simulink model "ctrl_HSMBObserver"  (R2015a)
settings: Solver=ode3  StartTime=0.0  StopTime=inf  FixedStep=0.01  RelTol=1e-3
values from neighbouring files (symbols this model uses):
  C = [C1;C2;C3;C4;C5;C6]    [initfile.m]    (also in thrustallocationQuadraticFixed.m)
  D = 3.0/100    (= 0.03)    [initfile.m]    (also in thrustallocationQuadraticFixed.m = 0.0411111111111)
  eps_c = 5    [initfile.m]
  epsilon = 0.5    [initfile.m]    (also in thrustallocationPseudo.m = u(10); thrustallocationQuadraticFixed.m = u(10))
  hd = c2d(H1,0.01,'foh')    [initfile.m]
  hd2 = c2d(H2,0.01,'zoh')    [initfile.m]
  I_s = 25000 /747225    (= 0.0334571246947)    [initfile.m]
  k_cc = 1    [initfile.m]
  K_omega = 0.3    [initfile.m]
  K_q1f = 0.0113    [initfile.m]
  K_q1r = K_q1f    (= 0.0113)    [initfile.m]
  K_q2f = 0.0117    [initfile.m]
  K_q2r = K_q2f    (= 0.0117)    [initfile.m]
  K_q3f = 0.0113    [initfile.m]
  K_q3r = K_q3f    (= 0.0113)    [initfile.m]
  K_q4f = 0.0169    [initfile.m]
  K_q4r = K_q4f    (= 0.0169)    [initfile.m]
  K_q5f = 0.0144    [initfile.m]
  K_q5r = K_q5f    (= 0.0144)    [initfile.m]
  K_q6f = 0.0168    [initfile.m]
  K_q6r = K_q6f    (= 0.0168)    [initfile.m]
  K_T1f = 0.3763    [initfile.m]
  K_T1r = K_T1f    (= 0.3763)    [initfile.m]
  K_T2f = 0.3901    [initfile.m]
  K_T2r = K_T2f    (= 0.3901)    [initfile.m]
  K_T3f = 0.3776    [initfile.m]
  K_T3r = K_T3f    (= 0.3776)    [initfile.m]
  K_T4f = 0.5641    [initfile.m]
  K_T4r = K_T4f    (= 0.5641)    [initfile.m]
  K_T5f = 0.4799    [initfile.m]
  K_T5r = K_T5f    (= 0.4799)    [initfile.m]
  K_T6f = 0.5588    [initfile.m]
  K_T6r = K_T6f    (= 0.5588)    [initfile.m]
  Kp = 3.3    [initfile.m]
  Max_Acceleration = 5    [initfile.m]
  Max_rotation = 12*sqrt(lambda)    [initfile.m]
  Max_thrust = 1.5    [initfile.m]
  Min_thrust = -0.8    [initfile.m]
  n_c = 5    [initfile.m]
  n_max = 152    [initfile.m]
  p_cc = 0.5    [initfile.m]
  pwm_thr1_backward = coeffvalues(ForceToPWM)    [initfile.m]
  pwm_thr1_forward = coeffvalues(ForceToPWM)    [initfile.m]
  pwm_thr2_backward = coeffvalues(ForceToPWM)    [initfile.m]
  pwm_thr2_forward = coeffvalues(ForceToPWM)    [initfile.m]
  pwm_thr3_backward = coeffvalues(ForceToPWM)    [initfile.m]
  pwm_thr3_forward = coeffvalues(ForceToPWM)    [initfile.m]
  pwm_thr4_backward = coeffvalues(ForceToPWM)    [initfile.m]
  pwm_thr4_forward = coeffvalues(ForceToPWM)    [initfile.m]
  pwm_thr5_backward = coeffvalues(ForceToPWM)    [initfile.m]
  pwm_thr5_forward = coeffvalues(ForceToPWM)    [initfile.m]
  pwm_thr6_backward = coeffvalues(ForceToPWM)    [initfile.m]
  pwm_thr6_forward = coeffvalues(ForceToPWM)    [initfile.m]
  Q_f0 = 0.3    [initfile.m]
  r_cc = 4    [initfile.m]
  Rho = Rho_m    (= 1000)    [initfile.m]
  ts = [-1 0]    [thrustallocationPseudo.m]    (also in thrustallocationQuadraticFixed.m)
undefined symbols (not defined in the file or in its folder): AFB, arm, Att, Control, Damping, FaultDet, Glob, Grip, IntActionType, Mass, NPO, Obs, Omg0_min, Q_max, ReferenceMdl, Sensor, Sim, SwLogic, tau, Thruster, Thruster_lock
libraries: dspmtrx3 x14, marine_gnc x11, simulink_extras x9, dspstat3 x9, simulink x9, dsparch4 x6, dspspect3 x6
(part 2 of 7)

== system ctrl_HSMBObserver/Data Logging ==
  eta_m : Inport
  eta_m_ideal : Inport  Port=2
  rate_m : Inport  Port=3
  acc_m : Inport  Port=4
  tau_c : Inport  Port=5
  tau_ca : Inport  Port=6
  angle_c : Inport  Port=7
  thrust_c : Inport  Port=8
  pwm_c : Inport  Port=9
  reference : Inport  Port=10
  controller : Inport  Port=11
  observer : Inport  Port=12
  fault : Inport  Port=13
  hat_wp : Inport  Port=14
  logic : Inport  Port=15
  PDF_control : Inport  Port=16
  PDF_reference : Inport  Port=17
  Mux : Mux  Inputs=17
  To File : ToFile  Filename=HSMBObserver.mat  MatrixName=data  SampleTime=0.01
  wires:
  eta_m/1 -> Mux/1
  Mux/1 -> To File/1
  eta_m_ideal/1 -> Mux/2
  rate_m/1 -> Mux/3
  acc_m/1 -> Mux/4
  tau_c/1 -> Mux/5
  angle_c/1 -> Mux/7
  thrust_c/1 -> Mux/8
  pwm_c/1 -> Mux/9
  tau_ca/1 -> Mux/6
  reference/1 -> Mux/10
  controller/1 -> Mux/11
  observer/1 -> Mux/12
  fault/1 -> Mux/13
  hat_wp/1 -> Mux/14
  logic/1 -> Mux/15
  PDF_control/1 -> Mux/16
  PDF_reference/1 -> Mux/17

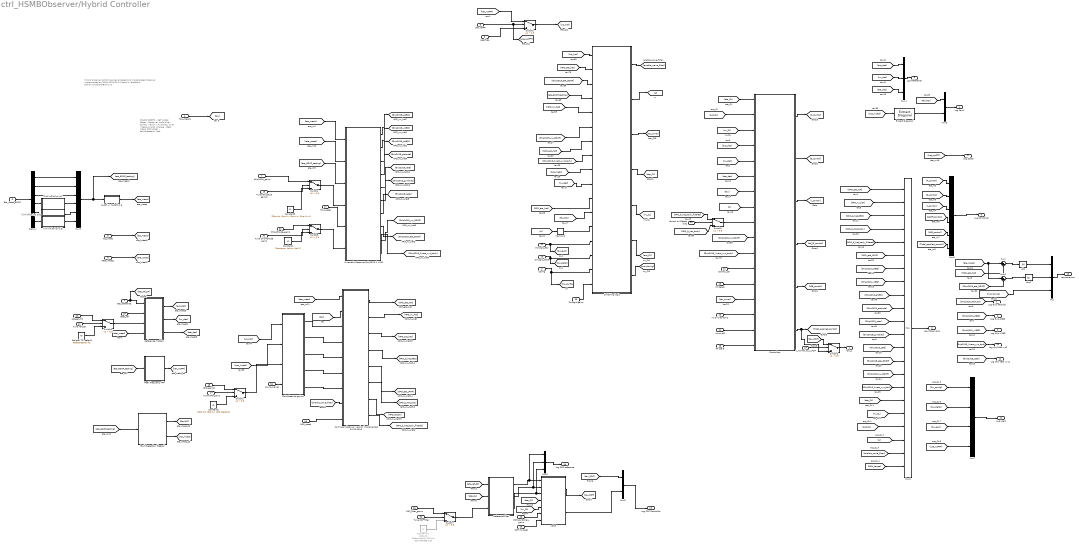
== system ctrl_HSMBObserver/Hybrid Controller ==
  note: Hybrid observer combining signal-based and model-based observer
      | Implemented on CSAD 2016-12-14
      | Astrid H. Brodtkorb astrid.h.brodtkorb@ntnu.no
  note: COLOR CODES:
      | 	- Ref model: Green
      | 	- Observer: Light blue
      | 	- Control: Yellow
      | 	- Hybrid/CL: Cyan
      | 	- Measurments: Orange
      | 	- Ideal meas: Dark green
      | 	- FaultDetection: Red
  Eta_reference : Inport
  Config : Inport  Port=2
  Eta_meas_6DOF : Inport  Port=3
  Tau_meas1 : Inport  Port=4
  Acc_meas : Inport  Port=5
  Rate_meas1 : Inport  Port=6
  Grip2015_gains : Inport  Port=7
  Use wpFFT : Inport  Port=8
  peakfreq : Inport  Port=9
  SwLogic_delta : Inport  Port=10
  SwLogic_eps : Inport  Port=11
  Control_par : Inport  Port=12
  Int Reset : Inport  Port=13
  Tune NPO gains : Inport  Port=14
  NPO_gains1 : Inport  Port=15
  Tune Grip2015 gains1 : Inport  Port=16
  Grip_reset : Inport  Port=17
  NPO_reset : Inport  Port=18
  reset_ref : Inport  Port=19
  ref_gen_TC : Inport  Port=20
  Tune ref gen : Inport  Port=21
  Normal or filtered bias : Inport  Port=22
  Int or bias comp : Inport  Port=23
  Int on/off : Inport  Port=24
  ref scale : Inport  Port=25
  PDF_filter_gains : Inport  Port=26
  u_normal_or_u_PDF : Inport  Port=27
  PDF_controller_gains : Inport  Port=28
  PDF int reset : Inport  Port=29
  Tune PDF filter : Inport  Port=30
  GripAttitude_gains : Inport  Port=31
  Tune GripAttitude gains : Inport  Port=32
  SwLogic.gains : Inport  Port=33
  K2_no_waves : Inport  Port=34
  6_dof --> 3_dof1,2,6 : Subsystem
  Abs : Abs
  Abs1 : Abs
  Calc observer gains1 : Subsystem  mask{lmb=Obs.NPO.lmb, k=Obs.NPO.k, zeta=Obs.NPO.damp}
      mask prompts: lmb "Control.VessObs.lmb{i}=lmb"; k "Control.VessObs.k{i}=k"; zeta "Control.VessObs.damp{i}=zeta"
  Constant1 : Constant  Value=[Att.sigma, Att.Kp, Att.Ki]
  Constant2 : Constant  Value=[NPO.K3, NPO.K4, NPO.scaleK2]
  Constant3 : Constant  Value=[Grip.Kp, Grip.Kv, Grip.Kxi, Grip.Kvvr]
  Controllers : Subsystem
  Demux : Demux  Outputs=6
  Extract Diagonal : dspmtrx3/Extract Diagonal
  Fault Detection (freeze) : Subsystem
  Kinematic Observer Grip2015 + VVR1 : Subsystem
  Memory2 : Memory  X0=Obs.Initial
  Mux : Mux  Inputs=3
  Mux2 : Mux  Inputs=6
  Mux3 : Mux  Inputs=2
  Mux4 : Mux  Inputs=3
  Mux5 : Mux  Inputs=6
  Mux6 : Mux  Inputs=22
  Mux7 : Mux
  Mux8 : Mux  Inputs=2
  Mux9 : Mux  Inputs=3
  "Nonlinear observer, version implemented 04.26.2016" : Subsystem
  Peak Frequency FFT : Subsystem
  "Ref gen TC, default" : Constant  Value=ReferenceMdl.TC
  "Ref gen TC, default1" : Constant  Commented=on  Value=ReferenceMdl.PDF.Par
  Reference filter : Subsystem
  Reference model2 : Subsystem
  Sum : Sum  Inputs=|+-
  Sum1 : Sum  Inputs=|+-
  Switch{1..8} (8 alike) : Switch  Criteria=u2 > Threshold  Threshold=0.5
  Switching logic : Subsystem
  "[-inf inf] to [-pi pi]" : Subsystem  AncestorBlock=marine_gnc/Utilities/Math Operations/[-inf inf] to [-pi pi]  mask([-inf inf] to [-pi pi]){}
      mask help: Converts an angle in rad to (-pi pi)
  "[-inf inf] to [-pi pi]1" : Subsystem  AncestorBlock=marine_gnc/Utilities/Math Operations/[-inf inf] to [-pi pi]  mask([-inf inf] to [-pi pi]){}
      mask help: Converts an angle in rad to (-pi pi)
  "[-inf inf] to [-pi pi]2" : Subsystem  AncestorBlock=marine_gnc/Utilities/Math Operations/[-inf inf] to [-pi pi]  mask([-inf inf] to [-pi pi]){}
      mask help: Converts an angle in rad to (-pi pi)
  nPDF : Subsystem
  tau_c : Outport
  Log Observers1 : Outport  Port=2
  Log Reference : Outport  Port=3
  Log Fault : Outport  Port=4
  Log SSest : Outport  Port=5
  Log Controller : Outport  Port=6
  Log Grip attitude : Outport  Port=7
  Log Grip pNED : Outport  Port=8
  Log Grip vNED : Outport  Port=9
  Log Grip acc xyz2 : Outport  Port=10
  Log Grip zeta xyz1 : Outport  Port=11
  Log Logic : Outport  Port=12
  Log PDF Controller : Outport  Port=13
  Log PDF reference : Outport  Port=14
  Log est errors : Outport  Port=15
  wires:
  Peak Frequency FFT/1(hat_wp) -> [hat_wpFFT]
  [eta_6DOF_testing] -> Kinematic Observer Grip2015 + VVR1/3(Eta_meas)
  [acc_meas] -> Kinematic Observer Grip2015 + VVR1/1(Acc_meas)
  Kinematic Observer Grip2015 + VVR1/2(vNED_hat) -> [Grip2015_vNED]  "Grip_nu_hat"
  Kinematic Observer Grip2015 + VVR1/3(aNED_hat) -> [Grip2015_aNED]  "Grip_acc_hat"
  Kinematic Observer Grip2015 + VVR1/1(pNED_hat) -> [Grip2015_pNED]  "Grip_eta_hat"
  Kinematic Observer Grip2015 + VVR1/10(Lin acc_xyz_body) -> [Grip2015_linacc_xyz_body]  "Grip_linacc_xy_body"
  6_dof --> 3_dof1,2,6/1(3DOF) -> [eta_meas]
  Eta_reference/1 -> Reference model2/1(Eta ref), [eta_ref_SP]
  Tau_meas1/1 -> [tau]
  [eta_6DOF_testing] -> Peak Frequency FFT/1(Eta_6DOF)
  Reference model2/1(Acc_des) -> [acc_des]
  Reference model2/2(Nu_des) -> [nu_des]
  Reference model2/3(Eta_des) -> [eta_des]
  Mux4/1 -> Log Reference/1
  [acc_des] -> Mux4/1  "acc_des"
  [nu_des] -> Mux4/2  "nu_des"
  [eta_des] -> Mux4/3  "eta_des"
  Mux3/1 -> Log Fault/1
  [FaultID] -> Mux3/1
  [pos_inject] -> Extract Diagonal/1
  [hat_wpFFT] -> Log SSest/1  "hat_wpFFT"
  Mux6/1 -> Log Observers1/1
  Switch2/1 -> [wp_hat]
  [hat_wpFFT] -> Switch2/1
  Use wpFFT/1 -> [use_wpFFT], Switch2/2
  Mux5/1 -> Log Controller/1
  [eta_6DOF_testing] -> Fault Detection (freeze)/1(Eta_6DOFmeas)
  Fault Detection (freeze)/1(fault) -> [FaultID]
  Fault Detection (freeze)/2(pos_injection) -> [pos_inject]
  [wp_hat] -> Switching logic/1(wp_hat)
  Switching logic/4(eta_CL) -> [eta_CL]  "eta_CL"
  [NPO_eta_hat] -> Switching logic/2(NPO_eta_hat)
  [eta_6DOF_testing] -> Switching logic/4(eta_meas_testing)
  [Grip2015_nu_3DOF] -> Switching logic/6(Grip_nu_hat)
  [Grip2015_linacc_xyz_body] -> Switching logic/8(Grip_acc_hat)
  [NPO_acc_hat] -> Switching logic/7(NPO_acc_hat)
  [NPO_eta_hat] -> Switching logic/11(eta_hat_NPO_LFWF)
  [FaultID] -> Switching logic/12(Fault_Detection)
  Switching logic/1(enable wave filter) -> [enable_wave_filter]  "enable_wavefilter"
  [q] -> Memory2/1
  Memory2/1 -> Switching logic/13(q_current)
  [Grip2015_eta_3DOF] -> Switching logic/3(Grip_eta_hat)
  [nu_des] -> Switching logic/10(nu desired)
  Switching logic/5(nu_CL) -> [nu_CL]
  Switching logic/6(acc_CL) -> [acc_CL]
  Switching logic/2(q) -> [q]  "q"
  Config/1 -> [Sw_config], Switching logic/16(CONFIG)
  SwLogic_delta/1 -> [Sw_delta], Switching logic/15(SwLogic.delta1)
  SwLogic_eps/1 -> [Sw_eps], Switching logic/14(SwLogic.eps)
  [nu_des] -> Controllers/5(Nu_des)
  [eta_des] -> Controllers/6(Eta_des)
  [q] -> Controllers/8(q)
  [tau] -> Controllers/7(tau)
  [acc_des] -> Controllers/4(acc_des)
  [acc_CL] -> Controllers/2(Acc_est_xyz)
  Switch3/1 -> Controllers/9(b_hat_body)
  [eta_CL] -> Controllers/1(Eta)
  [nu_CL] -> Controllers/3(Nu)
  [Grip2015_nu_3DOF] -> Controllers/10(Grip_nu_LFWF)
  [Grip2015_linacc_xyz_body] -> Controllers/11(Grip_acc_LFWF_xyz)
  [NPO_b_hat_body] -> Switch3/3
  [NPO_b_hat_body_filtered] -> Switch3/1
  Normal or filtered bias/1 -> Switch3/2
  Switching logic/3(tau_timer) -> [tau_timer]
  Control_par/1 -> Controllers/12(Control_par)
  Int Reset/1 -> Controllers/13(int_reset)
  [tau_timer] -> Controllers/14(tau_timer)
  Controllers/3(I_control) -> [I_control]  "I_control"
  Controllers/2(D_control) -> [D_control]  "D_control"
  Controllers/1(P_control) -> [P_control]  "P_control"
  Controllers/4(ref_FF_control) -> [ref_FF_control]  "ref_FF_conrol"
  Controllers/5(AFB_control) -> [AFB_control]  "AFB_control"
  Controllers/6(Total_applied_control) -> Switch6/3, [Total_applied_control]  "total_applied_control"
  [AFB_control] -> Mux5/5
  [Total_applied_control] -> Mux5/6
  [D_control] -> Mux5/2
  [I_control] -> Mux5/3
  [ref_FF_control] -> Mux5/4
  [P_control] -> Mux5/1
  Calc observer gains1/2(K2(w_1)) -> "Nonlinear observer, version implemented 04.26.2016"/4(K2)
  Calc observer gains1/5(K4) -> "Nonlinear observer, version implemented 04.26.2016"/7(K5)
  [eta_meas] -> "Nonlinear observer, version implemented 04.26.2016"/1(Eta_meas)
  Calc observer gains1/1(K1(w_p)) -> "Nonlinear observer, version implemented 04.26.2016"/3(K1)
  Calc observer gains1/4(K3min) -> "Nonlinear observer, version implemented 04.26.2016"/6(K3)
  [tau] -> "Nonlinear observer, version implemented 04.26.2016"/2(Tau)
  "Nonlinear observer, version implemented 04.26.2016"/1(Eta_hat) -> [NPO_eta_hat]  "NPO_eta_hat"
  "Nonlinear observer, version implemented 04.26.2016"/2(Nu_hat) -> [NPO_nu_hat]  "NPO_nu_hat"
  "Nonlinear observer, version implemented 04.26.2016"/4(b_hat_NED) -> [NPO_b_hat_NED]  "NPO_b_hat_NED"
  [wp_hat] -> Calc observer gains1/1(w_p)
  [pos_inject] -> Calc observer gains1/2(pos_injection)
  "Nonlinear observer, version implemented 04.26.2016"/5(Eta_LFWF) -> [NPO_eta_LFWF]  "NPO_eta_LFWF"
  "Nonlinear observer, version implemented 04.26.2016"/3(Acc_hat) -> [NPO_acc_hat]  "NPO_acc_hat"
  Calc observer gains1/3(Aw(w_p)) -> "Nonlinear observer, version implemented 04.26.2016"/5(Aw)
  "Nonlinear observer, version implemented 04.26.2016"/6(b_hat_body) -> [NPO_b_hat_body]  "NPO_b_hat_body"
  [enable_wave_filter] -> "Nonlinear observer, version implemented 04.26.2016"/8(Sim Wavefilter)
  [NPO_eta_hat] -> Mux6/1
  [NPO_nu_hat] -> Switching logic/5(NPO_nu_hat)
  Demux/6 -> "[-inf inf] to [-pi pi]2"/1(x [-inf inf])
  Demux/5 -> "[-inf inf] to [-pi pi]1"/1(x [-inf inf])
  Demux/4 -> "[-inf inf] to [-pi pi]"/1(x [-inf inf])
  "[-inf inf] to [-pi pi]2"/1(y [-pi pi]) -> Mux2/6
  "[-inf inf] to [-pi pi]1"/1(y [-pi pi]) -> Mux2/5
  "[-inf inf] to [-pi pi]"/1(y [-pi pi]) -> Mux2/4
  Demux/3 -> Mux2/3
  Demux/2 -> Mux2/2
  Demux/1 -> Mux2/1
  Eta_meas_6DOF/1 -> Demux/1
  Mux2/1 -> 6_dof --> 3_dof1,2,6/1(6DOF), [eta_6DOF_testing]
  "Nonlinear observer, version implemented 04.26.2016"/7(kappa) -> [NPO_kappa]  "NPO_kappa"
  "Nonlinear observer, version implemented 04.26.2016"/8(b_hat_body_filtered) -> [NPO_b_hat_body_filtered]
  Tune NPO gains/1 -> Switch1/2
  Tune Grip2015 gains1/1 -> Switch4/2
  Constant3/1 -> Switch4/3
  Grip_reset/1 -> Kinematic Observer Grip2015 + VVR1/5(Grip_reset)
  NPO_reset/1 -> "Nonlinear observer, version implemented 04.26.2016"/9(reset_NPO)
  Kinematic Observer Grip2015 + VVR1/7(zeta) -> [Grip2015_zeta]
  [Grip2015_gyrobias] -> Mux6/12
  [Grip2015_pNED] -> Log Grip pNED/1
  [Grip2015_vNED] -> Log Grip vNED/1
  [Grip2015_zeta] -> Log Grip zeta xyz1/1
  [Grip2015_linacc_xyz_body] -> Log Grip acc xyz2/1
  [NPO_nu_hat] -> Mux6/2
  [NPO_b_hat_NED] -> Mux6/3
  [NPO_b_hat_body] -> Mux6/4
  [NPO_b_hat_body_filtered] -> Mux6/5
  [Grip2015_rate] -> Mux6/11
  [Grip2015_attitude] -> Mux6/10
  [Grip2015_aNED] -> Mux6/9
  [Grip2015_vNED] -> Mux6/8
  [Grip2015_pNED] -> Mux6/7
  [NPO_eta_LFWF] -> Mux6/6  "NPO_eta_LFWF"
  Extract Diagonal/1 -> Mux3/2
  Grip2015_gains/1 -> Switch4/1
  Mux7/1 -> Log Logic/1
  [Sw_config] -> Mux7/1
  [Sw_delta] -> Mux7/2
  [Sw_eps] -> Mux7/3
  [use_wpFFT] -> Mux7/4
  Switch1/1 -> Calc observer gains1/3(NPO_gains)
  Constant2/1 -> Switch1/3
  NPO_gains1/1 -> Switch1/1
  [eta_meas] -> Reference model2/4(Eta meas)
  reset_ref/1 -> Reference model2/2(reset_ref)
  Tune ref gen/1 -> Switch5/2
  "Ref gen TC, default"/1 -> Switch5/3
  ref_gen_TC/1 -> Switch5/1
  Switch5/1 -> Reference model2/3(Ref_gen TC)
  Int or bias comp/1 -> Controllers/15(Int or bias comp)
  Int on/off/1 -> Controllers/16(Int on/off)
  peakfreq/1 -> Switch2/3
  ref scale/1 -> Controllers/17(ref_scale)
  Reference filter/3(v_dd_f) -> Mux9/3, nPDF/3(v_dd)
  Reference filter/2(v_d_f) -> Mux9/2, nPDF/2(v_d)
  Reference filter/1(eta_d_f) -> Mux9/1, nPDF/1(eta_d)
  [eta_ref_SP] -> Reference filter/1(eta_d)
  [eta_CL] -> Reference filter/2(eta)
  [eta_CL] -> nPDF/4(eta)
  [nu_CL] -> nPDF/5(nu)
  nPDF/1(tau) -> [tau_PDF]
  [tau_PDF] -> Switch6/1
  u_normal_or_u_PDF/1 -> Switch6/2
  Switch6/1 -> tau_c/1
  PDF_controller_gains/1 -> nPDF/6(PDF controller gains)
  PDF int reset/1 -> nPDF/7(int_reset)
  Tune PDF filter/1 -> Switch7/2
  "Ref gen TC, default1"/1 -> Switch7/3
  PDF_filter_gains/1 -> Switch7/1
  Switch7/1 -> Reference filter/3(PDF filter gains)
  Mux8/1 -> Log PDF Controller/1
  [tau_PDF] -> Mux8/1
  nPDF/2(Iaction_NED_PDF) -> Mux8/2
  Mux9/1 -> Log PDF reference/1
  Rate_meas1/1 -> [rate_meas]
  [rate_meas] -> Kinematic Observer Grip2015 + VVR1/2(Ang_rate_meas)
  Kinematic Observer Grip2015 + VVR1/8(eta_3DOF) -> [Grip2015_eta_3DOF]
  Kinematic Observer Grip2015 + VVR1/9(nu_3DOF) -> [Grip2015_nu_3DOF]
  Kinematic Observer Grip2015 + VVR1/4(attitude hat) -> [Grip2015_attitude]
  Kinematic Observer Grip2015 + VVR1/5(angular_rate hat) -> [Grip2015_rate]
  Kinematic Observer Grip2015 + VVR1/6(gyro bias hat) -> [Grip2015_gyrobias]
  [Grip2015_attitude] -> Log Grip attitude/1
  [NPO_kappa] -> Mux6/22
  [enable_wave_filter] -> Mux6/21
  [q] -> Mux6/20
  [acc_CL] -> Mux6/19
  [nu_CL] -> Mux6/18
  [eta_CL] -> Mux6/17
  [Grip2015_linacc_xyz_body] -> Mux6/16
  [Grip2015_nu_3DOF] -> Mux6/15
  [Grip2015_eta_3DOF] -> Mux6/14
  [Grip2015_zeta] -> Mux6/13
  Tune GripAttitude gains/1 -> Switch8/2
  Constant1/1 -> Switch8/3
  GripAttitude_gains/1 -> Switch8/1
  [acc_meas] -> Switching logic/9(acc_meas)
  Acc_meas/1 -> [acc_meas]
  Switch4/1 -> Kinematic Observer Grip2015 + VVR1/4(Grip2015_gains)
  Switch8/1 -> Kinematic Observer Grip2015 + VVR1/6(GripAttitude_gains1)
  SwLogic.gains/1 -> Switching logic/17(SwLogic.gains)
  Mux/1 -> Log est errors/1
  [eta_meas] -> Sum1/1, Sum/1
  [NPO_eta_hat] -> Sum/2
  [Grip2015_eta_3DOF] -> Sum1/2
  Sum/1 -> Abs/1
  Sum1/1 -> Abs1/1
  [monitoring] -> Mux/3
  Switching logic/7(monitoring) -> [monitoring]
  K2_no_waves/1 -> Calc observer gains1/4(K2_no_waves)
  Abs/1 -> Mux/1
  Abs1/1 -> Mux/2

== system ctrl_HSMBObserver/IMU frame to body frame ==
  note: Multiply acceleration to get a RH coordinate system. The angles are already in a RH coordinate system.
      | Then rotate the IMU axes to correspond with the ship axes. This is done by making a 180 deg rotation about the y-axis.
      | J1 = diag(-1, 1, -1), J2 = diag(1, 1, -1)
      | AHBrodtkorb astrid.h.brodtkorb@ntnu.no
  Acc IMU : Inport
  Rate : Inport  Port=2
  Demux : Demux  Outputs=3
  Demux1 : Demux  Outputs=3
  G to ms2 : Gain  Gain=9.81
  Mux1 : Mux  Inputs=3
  Mux2 : Mux  Inputs=3
  Static bias compensation test 18 : Constant  Value=[-0.0082, 0.0136, 0.0038]'
  Static bias compensation1 : Constant  Value=[-0.0023, -0.0068, 0.0047]'
  Static bias compensation2 logfile 19.dec : Constant  Value=[-9.9102e-4, 0.0024031, -0.0010433]'
  Static bias compensation2 logfile 19.dec1 : Constant  Value=[-5.68e-5, -1.2316e-4, 4.4085e-4]'
  Sum{1..4} (4 alike) : Sum  Inputs=|+-
  To RH coord : Gain  Gain=-1
  To body coord1 : Gain  Gain=-1
  To body coord2 : Gain  Gain=-1
  To body coord4 : Gain  Gain=-1
  deg to rad : Gain  Gain=pi/180
  Acc_m : Outport
  Rate_m1 : Outport  Port=2
  wires:
  Sum4/1 -> Sum2/1
  Mux1/1 -> Sum4/1
  Acc IMU/1 -> G to ms2/1
  Rate/1 -> deg to rad/1
  G to ms2/1 -> To RH coord/1
  Demux/1 -> To body coord1/1
  Demux/3 -> To body coord2/1
  Demux/2 -> Mux1/2
  Sum1/1 -> Sum3/1
  To RH coord/1 -> Demux/1
  To body coord1/1 -> Mux1/1
  To body coord2/1 -> Mux1/3
  Demux1/3 -> To body coord4/1
  Demux1/2 -> Mux2/2
  Demux1/1 -> Mux2/1
  To body coord4/1 -> Mux2/3
  deg to rad/1 -> Demux1/1
  Mux2/1 -> Sum1/1
  Sum3/1 -> Rate_m1/1
  Sum2/1 -> Acc_m/1
  Static bias compensation test 18/1 -> Sum4/2
  Static bias compensation1/1 -> Sum1/2
  Static bias compensation2 logfile 19.dec/1 -> Sum2/2
  Static bias compensation2 logfile 19.dec1/1 -> Sum3/2

== system ctrl_HSMBObserver/Subsystem1 ==
  Calculated angles : Inport
  Demux : Demux  Outputs=6
  Mux : Mux  Inputs=6
  Saturation {1..6} (6 alike) : Saturate  UpperLimit=pi  LowerLimit=-pi
  Commanded angles : Outport
  wires:
  Calculated angles/1 -> Demux/1
  Demux/1 -> Saturation 1/1
  Demux/2 -> Saturation 2/1
  Demux/3 -> Saturation 3/1
  Demux/4 -> Saturation 4/1
  Demux/5 -> Saturation 5/1
  Demux/6 -> Saturation 6/1
  Mux/1 -> Commanded angles/1
  Saturation 1/1 -> Mux/1
  Saturation 6/1 -> Mux/6
  Saturation 5/1 -> Mux/5
  Saturation 2/1 -> Mux/2
  Saturation 3/1 -> Mux/3
  Saturation 4/1 -> Mux/4

== system ctrl_HSMBObserver/TA fixed thrusters, pseudoinverse ==
  tau : Inport
  MATLAB Function : MATLAB Function  TreatAsAtomicUnit=on
  X-position Thruster : Constant  Value=[Thruster.T1(1) Thruster.T2(1) Thruster.T3(1) Thruster.T4(1) Thruster.T5(1) Thruster.T6(1)]
  Y-position Thruster : Constant  Value=[Thruster.T1(2) Thruster.T2(2) Thruster.T3(2) Thruster.T4(2) Thruster.T5(2) Thruster.T6(2)]
  constant angle1 : Constant  Value=[Thruster.T1(3) Thruster.T2(3) Thruster.T3(3) Thruster.T4(3) Thruster.T5(3) Thruster.T6(3)]
  u_des : Outport
  wires:
  tau/1 -> MATLAB Function/1(tau_c)
  X-position Thruster/1 -> MATLAB Function/2(ThrusterPosX)
  Y-position Thruster/1 -> MATLAB Function/3(ThrusterPosY)
  constant angle1/1 -> MATLAB Function/4(alpha)
  MATLAB Function/1(u) -> u_des/1

== system ctrl_HSMBObserver/Thrust allocation1 ==
  tau : Inport
  Angles : Inport  Port=2
  "  Thrust calculated" : Selector  InputPortWidth=12  Indices=[7 8 9 10 11 12]
  " Angle calculated" : Selector  InputPortWidth=12  Indices=[1 2 3 4 5 6]
  C : Constant  Value=C
  Choosing Fixed / Azimuth angle : Switch  Threshold=1
  Constant : Constant  Value=Thruster_lock
  Constant to avoid singularities : Constant  Value=eps
  MATLAB Function : MATLAB Function  TreatAsAtomicUnit=on
  Mux : Mux  Inputs=3
  Mux2 : Mux  Inputs=2
  Optimal angle path and constraints on rotation speed : Subsystem  TreatAsAtomicUnit=on
  Radians to Degrees : simulink_extras/Transformations/Radians to Degrees
  X-position Thruster : Constant  Value=[Thruster.T1(1) Thruster.T2(1) Thruster.T3(1) Thruster.T4(1) Thruster.T5(1) Thruster.T6(1)]
  Y-position Thruster : Constant  Value=[Thruster.T1(2) Thruster.T2(2) Thruster.T3(2) Thruster.T4(2) Thruster.T5(2) Thruster.T6(2)]
  angle between [-180 180] : MATLAB Function  TreatAsAtomicUnit=on
  constant angle : Constant  Value=[Thruster.T1(3) Thruster.T2(3) Thruster.T3(3) Thruster.T4(3) Thruster.T5(3) Thruster.T6(3)]
  reset : S-Function  Priority=1  FunctionName=NIVeriStandIO  Parameters=width dtype portnum stime stype btype  mask(NI VeriStand Inport){portnum=1, width=-1, stime=-1, dtype=auto, stype=auto, btype=1}
      mask prompts: portnum "Port number:"; width "Port dimensions (-1 for dynamically sized):"; stime "Sample time (-1 for inherited):"; dtype "Data type:"; stype "Signal type:"; btype "Block type:"
      mask help: Use this inport on any level of nested subsystems to allow NI VeriStand software to map signals to it.
      mask init:
      | NIVeriStandIO_init;
      settings: CopyFcn=NIVeriStand_MDL_functions('', 'IO_copy');  DeleteFcn=NIVeriStand_MDL_functions('', 'IO_delete');  MoveFcn=set_param(gcb, 'Mask', 'on');
      mask Callback portnum: NIVeriStand_MDL_functions('', 'IO_setportnum');
      mask TypeOptions dtype: auto | double | single | int8 | uint8 | int16 | uint16 | int32 | uint32 | boolean
      mask Callback dtype: NIVeriStand_MDL_functions('', 'IO_booleansignal');
      mask TypeOptions stype: auto | real | complex
      mask Display:
      | patch([-x x], [-y y], [.90980 .81960 .32156]);
      | plot([xrad -x x xrad], [yrad -y y yrad]);
      | fprintf('NI In%d', portnum);
  u_d & angle : Outport
  wires:
  Constant to avoid singularities/1 -> Mux/3
  " Angle calculated"/1 -> Choosing Fixed / Azimuth angle/1
  Mux2/1 -> u_d & angle/1
  "  Thrust calculated"/1 -> Mux2/2
  tau/1 -> Mux/1
  Choosing Fixed / Azimuth angle/1 -> Optimal angle path and constraints on rotation speed/1(Desired Angle)
  Angles/1 -> angle between [-180 180]/1(angle)
  Optimal angle path and constraints on rotation speed/1(commanded Angle) -> Mux2/1
  constant angle/1 -> Optimal angle path and constraints on rotation speed/2("initial angle "), Choosing Fixed / Azimuth angle/3
  Radians to Degrees/1 -> Mux/2
  reset/1 -> Optimal angle path and constraints on rotation speed/3(reset)
  X-position Thruster/1 -> MATLAB Function/2(ThrusterPosX)
  Y-position Thruster/1 -> MATLAB Function/3(ThrusterPosY)
  C/1 -> MATLAB Function/4(C)
  MATLAB Function/1(sys) -> " Angle calculated"/1, "  Thrust calculated"/1
  Mux/1 -> MATLAB Function/1(u)
  angle between [-180 180]/1(y) -> Radians to Degrees/1
  Constant/1 -> Choosing Fixed / Azimuth angle/2

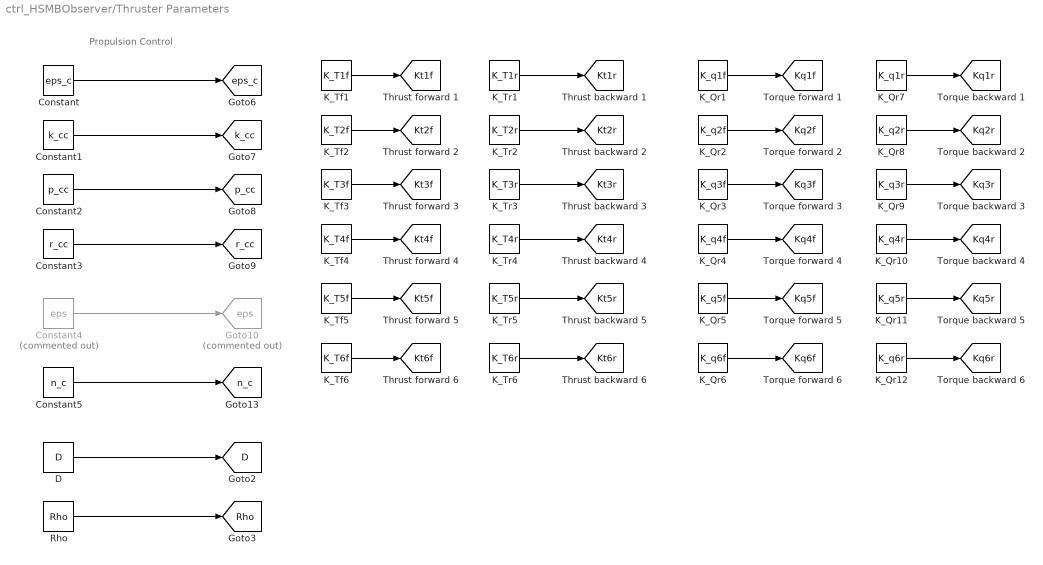
== system ctrl_HSMBObserver/Thruster Parameters  ==
  note: Propulsion Control
  Constant : Constant  Value=eps_c
  Constant1 : Constant  Value=k_cc
  Constant2 : Constant  Value=p_cc
  Constant3 : Constant  Value=r_cc
  Constant4 : Constant  Commented=on  Value=eps
  Constant5 : Constant  Value=n_c
  D : Constant  Value=D
  Goto10 : Goto  Commented=on  GotoTag=eps  TagVisibility=global
  K_Qr1 : Constant  Value=K_q1f
  K_Qr10 : Constant  Value=K_q4r
  K_Qr11 : Constant  Value=K_q5r
  K_Qr12 : Constant  Value=K_q6r
  K_Qr2 : Constant  Value=K_q2f
  K_Qr3 : Constant  Value=K_q3f
  K_Qr4 : Constant  Value=K_q4f
  K_Qr5 : Constant  Value=K_q5f
  K_Qr6 : Constant  Value=K_q6f
  K_Qr7 : Constant  Value=K_q1r
  K_Qr8 : Constant  Value=K_q2r
  K_Qr9 : Constant  Value=K_q3r
  K_Tf1 : Constant  Value=K_T1f
  K_Tf2 : Constant  Value=K_T2f
  K_Tf3 : Constant  Value=K_T3f
  K_Tf4 : Constant  Value=K_T4f
  K_Tf5 : Constant  Value=K_T5f
  K_Tf6 : Constant  Value=K_T6f
  K_Tr1 : Constant  Value=K_T1r
  K_Tr2 : Constant  Value=K_T2r
  K_Tr3 : Constant  Value=K_T3r
  K_Tr4 : Constant  Value=K_T4r
  K_Tr5 : Constant  Value=K_T5r
  K_Tr6 : Constant  Value=K_T6r
  Rho : Constant  Value=Rho
  tag scope: D=global, Kq1f=global, Kq1r=global, Kq2f=global, Kq2r=global, Kq3f=global, Kq3r=global, Kq4f=global, Kq4r=global, Kq5f=global, Kq5r=global, Kq6f=global, Kq6r=global, Kt1f=global, Kt1r=global, Kt2f=global, Kt2r=global, Kt3f=global, Kt3r=global, Kt4f=global, Kt4r=global, Kt5f=global, Kt5r=global, Kt6f=global, Kt6r=global, Rho=global, eps_c=global, k_cc=global, n_c=global, p_cc=global, r_cc=global
  wires:
  D/1 -> [D]
  Rho/1 -> [Rho]
  Constant/1 -> [eps_c]
  Constant1/1 -> [k_cc]
  Constant2/1 -> [p_cc]
  Constant3/1 -> [r_cc]
  Constant4/1 -> Goto10/1
  Constant5/1 -> [n_c]
  K_Tf1/1 -> [Kt1f]
  K_Tf6/1 -> [Kt6f]
  K_Tf5/1 -> [Kt5f]
  K_Tf4/1 -> [Kt4f]
  K_Tf3/1 -> [Kt3f]
  K_Tf2/1 -> [Kt2f]
  K_Tr1/1 -> [Kt1r]
  K_Tr6/1 -> [Kt6r]
  K_Tr5/1 -> [Kt5r]
  K_Tr4/1 -> [Kt4r]
  K_Tr2/1 -> [Kt2r]
  K_Tr3/1 -> [Kt3r]
  K_Qr1/1 -> [Kq1f]
  K_Qr2/1 -> [Kq2f]
  K_Qr3/1 -> [Kq3f]
  K_Qr4/1 -> [Kq4f]
  K_Qr5/1 -> [Kq5f]
  K_Qr6/1 -> [Kq6f]
  K_Qr7/1 -> [Kq1r]
  K_Qr8/1 -> [Kq2r]
  K_Qr9/1 -> [Kq3r]
  K_Qr10/1 -> [Kq4r]
  K_Qr11/1 -> [Kq5r]
  K_Qr12/1 -> [Kq6r]

== system ctrl_HSMBObserver/Thruster control  ==
  "Desired thrust and angle " : Inport
  Delay : Delay  DelayLength=1  InitialCondition=0
  Demux : Demux  Outputs=12
  Mapping shaft speed and thrust : Selector  InputPortWidth=12  Indices="[1 7 2  8 3 9 4 10 5 11 6 12]"
  Mux : Mux  Inputs=12
  Mux1 : Mux  Inputs=2
  Selecting Desired thrust1 : Selector  InputPortWidth=12  Indices=[7 8 9 10 11 12]
  Selecting actual angle : Selector  InputPortWidth=12  Indices=[1 2 3 4 5 6]
  Subsystem1 : Subsystem
  Thrust and Shaft speed mapped to PWM : Subsystem
  Thruster 1 : Subsystem
      settings: AttributesFormatString=%<MinAlgLoopOccurrences>
  Thruster 2 : Subsystem
      settings: AttributesFormatString=%<MinAlgLoopOccurrences>
  Thruster 3 : Subsystem
      settings: AttributesFormatString=%<MinAlgLoopOccurrences>
  Thruster 4 : Subsystem
      settings: AttributesFormatString=%<MinAlgLoopOccurrences>
  Thruster 5 : Subsystem
      settings: AttributesFormatString=%<MinAlgLoopOccurrences>
  Thruster 6 : Subsystem
      settings: AttributesFormatString=%<MinAlgLoopOccurrences>
  "Commanded pwm " : Outport
  Commanded angle : Outport  Port=2
  Commanded thrust : Outport  Port=3
  wires:
  Selecting actual angle/1 -> Subsystem1/1(Calculated angles)
  "Desired thrust and angle "/1 -> Selecting actual angle/1, Selecting Desired thrust1/1
  Subsystem1/1(Commanded angles) -> Commanded angle/1
  Thrust and Shaft speed mapped to PWM/1(pwm) -> "Commanded pwm "/1
  Thrust and Shaft speed mapped to PWM/2(Force) -> Commanded thrust/1
  Thrust and Shaft speed mapped to PWM/3("Shaft speed ") -> Delay/1
  Thruster 1/1("Commanded thrust ") -> Mux/1
  Mux/1 -> Thrust and Shaft speed mapped to PWM/1(Calculated thrust)
  Mux1/1 -> Mapping shaft speed and thrust/1
  Delay/1 -> Mux1/2
  Mapping shaft speed and thrust/1 -> Demux/1
  Thruster 1/2(Shaft speed) -> Mux/2
  Demux/2 -> Thruster 1/2(shaft speed)
  Demux/1 -> Thruster 1/1(Desired thrust 1)
  Thruster 2/1("Commanded thrust ") -> Mux/3
  Demux/3 -> Thruster 2/1(Desired thrust 1)
  Demux/4 -> Thruster 2/2(shaft speed)
  Demux/5 -> Thruster 3/1(Desired thrust 1)
  Demux/6 -> Thruster 3/2(shaft speed)
  Demux/7 -> Thruster 4/1(Desired thrust 1)
  Demux/8 -> Thruster 4/2(shaft speed)
  Demux/9 -> Thruster 5/1(Desired thrust 1)
  Demux/10 -> Thruster 5/2(shaft speed)
  Demux/11 -> Thruster 6/1(Desired thrust 1)
  Demux/12 -> Thruster 6/2(shaft speed)
  Thruster 2/2(Shaft speed) -> Mux/4
  Thruster 3/1("Commanded thrust ") -> Mux/5
  Thruster 3/2(Shaft speed) -> Mux/6
  Thruster 4/1("Commanded thrust ") -> Mux/7
  Thruster 4/2(Shaft speed) -> Mux/8
  Thruster 5/1("Commanded thrust ") -> Mux/9
  Thruster 5/2(Shaft speed) -> Mux/10
  Thruster 6/1("Commanded thrust ") -> Mux/11
  Thruster 6/2(Shaft speed) -> Mux/12
  Selecting Desired thrust1/1 -> Mux1/1

== system ctrl_HSMBObserver/Thruster measurment ==
  Mux1 : Mux  Inputs=6
  thr_angle_1 : S-Function  Priority=1  FunctionName=NIVeriStandIO  Parameters=width dtype portnum stime stype btype  mask(NI VeriStand Inport){portnum=1, width=-1, stime=-1, dtype=auto, stype=auto, btype=1}
      mask prompts: portnum "Port number:"; width "Port dimensions (-1 for dynamically sized):"; stime "Sample time (-1 for inherited):"; dtype "Data type:"; stype "Signal type:"; btype "Block type:"
      mask help: Use this inport on any level of nested subsystems to allow NI VeriStand software to map signals to it.
      mask init:
      | NIVeriStandIO_init;
      settings: CopyFcn=NIVeriStand_MDL_functions('', 'IO_copy');  DeleteFcn=NIVeriStand_MDL_functions('', 'IO_delete');  MoveFcn=set_param(gcb, 'Mask', 'on');
      mask Callback portnum: NIVeriStand_MDL_functions('', 'IO_setportnum');
      mask TypeOptions dtype: auto | double | single | int8 | uint8 | int16 | uint16 | int32 | uint32 | boolean
      mask Callback dtype: NIVeriStand_MDL_functions('', 'IO_booleansignal');
      mask TypeOptions stype: auto | real | complex
      mask Display:
      | patch([-x x], [-y y], [.90980 .81960 .32156]);
      | plot([xrad -x x xrad], [yrad -y y yrad]);
      | fprintf('NI In%d', portnum);
  thr_angle_2 : S-Function  Priority=2  FunctionName=NIVeriStandIO  Parameters=width dtype portnum stime stype btype  mask(NI VeriStand Inport){portnum=2, width=-1, stime=-1, dtype=auto, stype=auto, btype=1}
      mask prompts: portnum "Port number:"; width "Port dimensions (-1 for dynamically sized):"; stime "Sample time (-1 for inherited):"; dtype "Data type:"; stype "Signal type:"; btype "Block type:"
      mask help: Use this inport on any level of nested subsystems to allow NI VeriStand software to map signals to it.
      mask init:
      | NIVeriStandIO_init;
      settings: CopyFcn=NIVeriStand_MDL_functions('', 'IO_copy');  DeleteFcn=NIVeriStand_MDL_functions('', 'IO_delete');  MoveFcn=set_param(gcb, 'Mask', 'on');
      mask Callback portnum: NIVeriStand_MDL_functions('', 'IO_setportnum');
      mask TypeOptions dtype: auto | double | single | int8 | uint8 | int16 | uint16 | int32 | uint32 | boolean
      mask Callback dtype: NIVeriStand_MDL_functions('', 'IO_booleansignal');
      mask TypeOptions stype: auto | real | complex
      mask Display:
      | patch([-x x], [-y y], [.90980 .81960 .32156]);
      | plot([xrad -x x xrad], [yrad -y y yrad]);
      | fprintf('NI In%d', portnum);
  thr_angle_3 : S-Function  Priority=3  FunctionName=NIVeriStandIO  Parameters=width dtype portnum stime stype btype  mask(NI VeriStand Inport){portnum=3, width=-1, stime=-1, dtype=auto, stype=auto, btype=1}
      mask prompts: portnum "Port number:"; width "Port dimensions (-1 for dynamically sized):"; stime "Sample time (-1 for inherited):"; dtype "Data type:"; stype "Signal type:"; btype "Block type:"
      mask help: Use this inport on any level of nested subsystems to allow NI VeriStand software to map signals to it.
      mask init:
      | NIVeriStandIO_init;
      settings: CopyFcn=NIVeriStand_MDL_functions('', 'IO_copy');  DeleteFcn=NIVeriStand_MDL_functions('', 'IO_delete');  MoveFcn=set_param(gcb, 'Mask', 'on');
      mask Callback portnum: NIVeriStand_MDL_functions('', 'IO_setportnum');
      mask TypeOptions dtype: auto | double | single | int8 | uint8 | int16 | uint16 | int32 | uint32 | boolean
      mask Callback dtype: NIVeriStand_MDL_functions('', 'IO_booleansignal');
      mask TypeOptions stype: auto | real | complex
      mask Display:
      | patch([-x x], [-y y], [.90980 .81960 .32156]);
      | plot([xrad -x x xrad], [yrad -y y yrad]);
      | fprintf('NI In%d', portnum);
  thr_angle_4 : S-Function  Priority=4  FunctionName=NIVeriStandIO  Parameters=width dtype portnum stime stype btype  mask(NI VeriStand Inport){portnum=4, width=-1, stime=-1, dtype=auto, stype=auto, btype=1}
      mask prompts: portnum "Port number:"; width "Port dimensions (-1 for dynamically sized):"; stime "Sample time (-1 for inherited):"; dtype "Data type:"; stype "Signal type:"; btype "Block type:"
      mask help: Use this inport on any level of nested subsystems to allow NI VeriStand software to map signals to it.
      mask init:
      | NIVeriStandIO_init;
      settings: CopyFcn=NIVeriStand_MDL_functions('', 'IO_copy');  DeleteFcn=NIVeriStand_MDL_functions('', 'IO_delete');  MoveFcn=set_param(gcb, 'Mask', 'on');
      mask Callback portnum: NIVeriStand_MDL_functions('', 'IO_setportnum');
      mask TypeOptions dtype: auto | double | single | int8 | uint8 | int16 | uint16 | int32 | uint32 | boolean
      mask Callback dtype: NIVeriStand_MDL_functions('', 'IO_booleansignal');
      mask TypeOptions stype: auto | real | complex
      mask Display:
      | patch([-x x], [-y y], [.90980 .81960 .32156]);
      | plot([xrad -x x xrad], [yrad -y y yrad]);
      | fprintf('NI In%d', portnum);
  thr_angle_5 : S-Function  Priority=5  FunctionName=NIVeriStandIO  Parameters=width dtype portnum stime stype btype  mask(NI VeriStand Inport){portnum=5, width=-1, stime=-1, dtype=auto, stype=auto, btype=1}
      mask prompts: portnum "Port number:"; width "Port dimensions (-1 for dynamically sized):"; stime "Sample time (-1 for inherited):"; dtype "Data type:"; stype "Signal type:"; btype "Block type:"
      mask help: Use this inport on any level of nested subsystems to allow NI VeriStand software to map signals to it.
      mask init:
      | NIVeriStandIO_init;
      settings: CopyFcn=NIVeriStand_MDL_functions('', 'IO_copy');  DeleteFcn=NIVeriStand_MDL_functions('', 'IO_delete');  MoveFcn=set_param(gcb, 'Mask', 'on');
      mask Callback portnum: NIVeriStand_MDL_functions('', 'IO_setportnum');
      mask TypeOptions dtype: auto | double | single | int8 | uint8 | int16 | uint16 | int32 | uint32 | boolean
      mask Callback dtype: NIVeriStand_MDL_functions('', 'IO_booleansignal');
      mask TypeOptions stype: auto | real | complex
      mask Display:
      | patch([-x x], [-y y], [.90980 .81960 .32156]);
      | plot([xrad -x x xrad], [yrad -y y yrad]);
      | fprintf('NI In%d', portnum);
  thr_angle_6 : S-Function  Priority=6  FunctionName=NIVeriStandIO  Parameters=width dtype portnum stime stype btype  mask(NI VeriStand Inport){portnum=6, width=-1, stime=-1, dtype=auto, stype=auto, btype=1}
      mask prompts: portnum "Port number:"; width "Port dimensions (-1 for dynamically sized):"; stime "Sample time (-1 for inherited):"; dtype "Data type:"; stype "Signal type:"; btype "Block type:"
      mask help: Use this inport on any level of nested subsystems to allow NI VeriStand software to map signals to it.
      mask init:
      | NIVeriStandIO_init;
      settings: CopyFcn=NIVeriStand_MDL_functions('', 'IO_copy');  DeleteFcn=NIVeriStand_MDL_functions('', 'IO_delete');  MoveFcn=set_param(gcb, 'Mask', 'on');
      mask Callback portnum: NIVeriStand_MDL_functions('', 'IO_setportnum');
      mask TypeOptions dtype: auto | double | single | int8 | uint8 | int16 | uint16 | int32 | uint32 | boolean
      mask Callback dtype: NIVeriStand_MDL_functions('', 'IO_booleansignal');
      mask TypeOptions stype: auto | real | complex
      mask Display:
      | patch([-x x], [-y y], [.90980 .81960 .32156]);
      | plot([xrad -x x xrad], [yrad -y y yrad]);
      | fprintf('NI In%d', portnum);
  alpha_m : Outport
  wires:
  thr_angle_3/1 -> Mux1/3
  thr_angle_1/1 -> Mux1/1
  Mux1/1 -> alpha_m/1
  thr_angle_5/1 -> Mux1/5
  thr_angle_4/1 -> Mux1/4
  thr_angle_6/1 -> Mux1/6
  thr_angle_2/1 -> Mux1/2

== system ctrl_HSMBObserver/To meters and radians, noise and sampling ==
  In1 : Inport
  use noise : Inport  Port=2
  Degrees to Radians : simulink_extras/Transformations/Degrees to Radians
  Degrees to Radians1 : simulink_extras/Transformations/Degrees to Radians
  Degrees to Radians2 : simulink_extras/Transformations/Degrees to Radians
  Demux : Demux  Outputs=6
  Demux1 : Demux  Outputs=3
  Gain : Gain  Gain=1/1000
  Gain1 : Gain  Gain=1/1000
  Gain2 : Gain  Gain=1/1000
  Mux : Mux  Inputs=6
  Mux1 : Mux  Inputs=3
  Mux2 : Mux  Inputs=3
  Mux3 : Mux  Inputs=6
  SampleTime : Subsystem
  Sensor noise models : Subsystem  TreatAsAtomicUnit=on
  Sum : Sum  Inputs=|++
  Switch5 : Switch  Criteria=u2 > Threshold  Threshold=0.5
  "[-inf inf] to [-pi pi]1" : Subsystem  AncestorBlock=marine_gnc/Utilities/Math Operations/[-inf inf] to [-pi pi]  mask([-inf inf] to [-pi pi]){}
      mask help: Converts an angle in rad to (-pi pi)
  "[-inf inf] to [-pi pi]2" : Subsystem  AncestorBlock=marine_gnc/Utilities/Math Operations/[-inf inf] to [-pi pi]  mask([-inf inf] to [-pi pi]){}
      mask help: Converts an angle in rad to (-pi pi)
  "[-inf inf] to [-pi pi]3" : Subsystem  AncestorBlock=marine_gnc/Utilities/Math Operations/[-inf inf] to [-pi pi]  mask([-inf inf] to [-pi pi]){}
      mask help: Converts an angle in rad to (-pi pi)
  Eta : Outport
  eta_ideal : Outport  Port=2
  wires:
  Mux/1 -> Eta/1
  Demux/2 -> Gain/1
  Demux/1 -> Gain1/1
  Degrees to Radians/1 -> "[-inf inf] to [-pi pi]3"/1(x [-inf inf])
  Demux/6 -> Degrees to Radians/1
  Demux/5 -> Degrees to Radians1/1
  Degrees to Radians1/1 -> "[-inf inf] to [-pi pi]1"/1(x [-inf inf])
  Demux/4 -> Degrees to Radians2/1
  Degrees to Radians2/1 -> "[-inf inf] to [-pi pi]2"/1(x [-inf inf])
  Gain2/1 -> Mux3/3, Mux/3
  Demux/3 -> Gain2/1
  "[-inf inf] to [-pi pi]2"/1(y [-pi pi]) -> Mux3/4, Mux/4
  "[-inf inf] to [-pi pi]1"/1(y [-pi pi]) -> Mux3/5, Mux/5
  "[-inf inf] to [-pi pi]3"/1(y [-pi pi]) -> Mux2/3, Mux1/3, Mux3/6
  In1/1 -> Demux/1
  SampleTime/1(ReducedRates) -> Switch5/1
  Sensor noise models/1(Eta_noise) -> Sum/1
  Sum/1 -> SampleTime/1(Rate)
  use noise/1 -> Switch5/2
  Mux1/1 -> Sum/2
  Mux2/1 -> Switch5/3
  Switch5/1 -> Demux1/1
  Demux1/1 -> Mux/1
  Demux1/2 -> Mux/2
  Demux1/3 -> Mux/6
  Mux3/1 -> eta_ideal/1
  Gain1/1 -> Mux3/1, Mux2/1, Mux1/1
  Gain/1 -> Mux3/2, Mux2/2, Mux1/2

== system ctrl_HSMBObserver/To meters and radians2 ==
  In1 : Inport
  Degrees to Radians2 : simulink_extras/Transformations/Degrees to Radians
  Demux : Demux  Outputs=3
  Gain : Gain  Gain=1/1000
  Gain1 : Gain  Gain=1/1000
  Gain4 : Gain  Commented=on  Gain=-1
  Mux : Mux  Inputs=3
  "[-inf inf] to [-pi pi]2" : marine_gnc/Utilities/Math Operations/[-inf inf] to [-pi pi]
  Etad_3DOF : Outport
  wires:
  Mux/1 -> Etad_3DOF/1
  Demux/2 -> Gain/1
  Demux/1 -> Gain1/1
  Degrees to Radians2/1 -> "[-inf inf] to [-pi pi]2"/1
  In1/1 -> Demux/1
  Gain/1 -> Mux/2
  Gain1/1 -> Mux/1
  Demux/3 -> Degrees to Radians2/1
  "[-inf inf] to [-pi pi]2"/1 -> Mux/3

== system ctrl_HSMBObserver/Veristand to IMU frame ==
  note: The measurements into Veristand do not correspond with the IMU axis.
      | Here the measurements are transformed to the IMU coordinate system.
      | AHBrodtkorb astrid.h.brodtkorb@ntnu.no
  In1 : Inport
  In2 : Inport  Port=2
  Demux3 : Demux  Outputs=3
  Demux4 : Demux  Outputs=3
  Mux1 : Mux  Inputs=3
  Mux2 : Mux  Inputs=3
  millig to g : Gain  Gain=0.001
  minus 1 : Gain  Gain=-1
  to 0.05 deg : Gain  Gain=1000
  to deg : Gain  Gain=0.05
  to millig : Gain  Gain=1/0.05
  Out1 : Outport
  Out2 : Outport  Port=2
  wires:
  In2/1 -> Demux4/1
  In1/1 -> Demux3/1
  Mux2/1 -> Out1/1
  Mux1/1 -> Out2/1
  Demux4/3 -> to millig/1
  Demux3/1 -> Mux2/2
  Demux3/2 -> Mux2/3
  Demux4/1 -> Mux1/2
  Demux4/2 -> Mux1/3
  Demux3/3 -> minus 1/1
  to millig/1 -> millig to g/1
  millig to g/1 -> Mux2/1
  to 0.05 deg/1 -> to deg/1
  to deg/1 -> Mux1/1
  minus 1/1 -> to 0.05 deg/1

== system ctrl_HSMBObserver/Hybrid Controller/6_dof --> 3_dof1,2,6 ==
  note: Extracting surge and sway
      | acceleration for measurement
      | TD Nguyen, 2005
  6DOF : Inport
  Selector : Selector  InputPortWidth=6  Indices=[1 2 6]
  3DOF : Outport
  wires:
  Selector/1 -> 3DOF/1
  6DOF/1 -> Selector/1

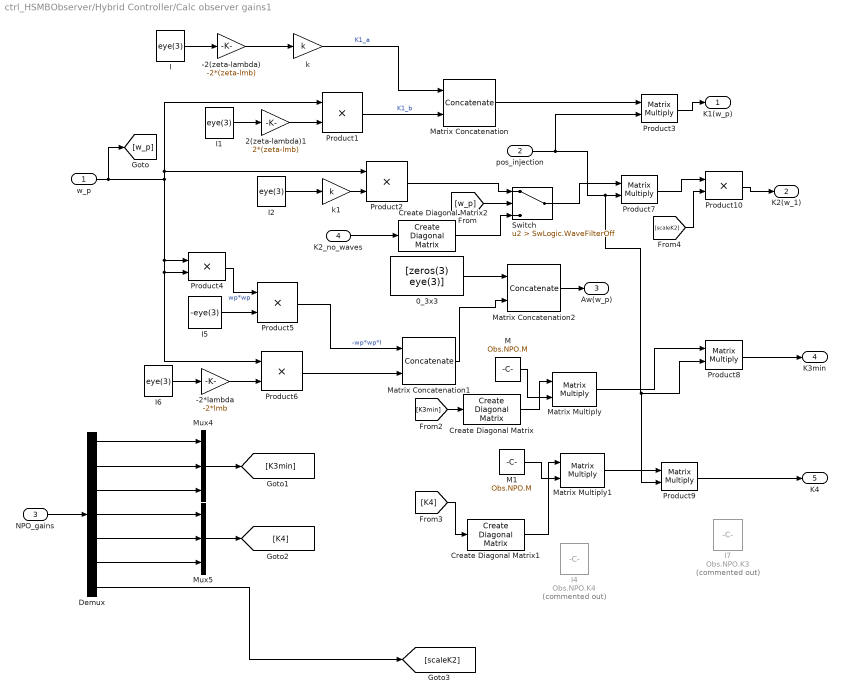
== system ctrl_HSMBObserver/Hybrid Controller/Calc observer gains1 ==
  w_p : Inport
  pos_injection : Inport  Port=2
  NPO_gains : Inport  Port=3
  K2_no_waves : Inport  Port=4
  -2(zeta-lambda) : Gain  Gain=-2*(zeta-lmb)  SaturateOnIntegerOverflow=on  OutDataTypeStr=Inherit: Same as input  ParamDataTypeStr=Inherit: Same as input
  -2*lambda : Gain  Gain=-2*lmb  SaturateOnIntegerOverflow=on  OutDataTypeStr=Inherit: Same as input  ParamDataTypeStr=Inherit: Same as input
  0_3x3 : Constant  Value=[zeros(3) eye(3)]
  2(zeta-lambda)1 : Gain  Gain=2*(zeta-lmb)  SaturateOnIntegerOverflow=on  OutDataTypeStr=Inherit: Same as input  ParamDataTypeStr=Inherit: Same as input
  Create Diagonal Matrix : dspmtrx3/Create Diagonal Matrix
  Create Diagonal Matrix1 : dspmtrx3/Create Diagonal Matrix
  Create Diagonal Matrix2 : dspmtrx3/Create Diagonal Matrix
  Demux : Demux  Outputs=7
  I{,1..2,6} (4 alike) : Constant  Value=eye(3)
  I4 : Constant  Commented=on  Value=Obs.NPO.K4
  I5 : Constant  Value=-eye(3)
  I7 : Constant  Commented=on  Value=Obs.NPO.K3
  M : Constant  Value=Obs.NPO.M
  M1 : Constant  Value=Obs.NPO.M
  Matrix Concatenation : Concatenate  Mode=Multidimensional array
  Matrix Concatenation1 : Concatenate  Mode=Multidimensional array  ConcatenateDimension=2
  Matrix Concatenation2 : Concatenate  Mode=Multidimensional array
  Matrix Multiply : Product  Multiplication=Matrix(*)
  Matrix Multiply1 : Product  Multiplication=Matrix(*)
  Mux4 : Mux  Inputs=3
  Mux5 : Mux  Inputs=3
  Product{1..2,4..6,10} (6 alike) : Product  SaturateOnIntegerOverflow=on  OutDataTypeStr=Inherit: Same as first input
  Product{3,7..9} (4 alike) : Product  Multiplication=Matrix(*)  SaturateOnIntegerOverflow=on  OutDataTypeStr=Inherit: Same as first input
  Switch : Switch  Criteria=u2 > Threshold  Threshold=SwLogic.WaveFilterOff
  k : Gain  Gain=k  SaturateOnIntegerOverflow=on  OutDataTypeStr=Inherit: Same as input  ParamDataTypeStr=Inherit: Same as input
  k1 : Gain  Gain=k  SaturateOnIntegerOverflow=on  OutDataTypeStr=Inherit: Same as input  ParamDataTypeStr=Inherit: Same as input
  K1(w_p) : Outport
  K2(w_1) : Outport  Port=2
  Aw(w_p) : Outport  Port=3
  K3min : Outport  Port=4
  K4 : Outport  Port=5
  wires:
  Matrix Concatenation2/1 -> Aw(w_p)/1
  0_3x3/1 -> Matrix Concatenation2/1
  Matrix Concatenation1/1 -> Matrix Concatenation2/2
  Product6/1 -> Matrix Concatenation1/2
  -2*lambda/1 -> Product6/2
  I6/1 -> -2*lambda/1
  Product5/1 -> Matrix Concatenation1/1  "-wp*wp*I"
  I5/1 -> Product5/2
  Product4/1 -> Product5/1  "wp*wp"
  k/1 -> Matrix Concatenation/1  "K1_a"
  Product1/1 -> Matrix Concatenation/2  "K1_b"
  2(zeta-lambda)1/1 -> Product1/2
  I1/1 -> 2(zeta-lambda)1/1
  -2(zeta-lambda)/1 -> k/1
  I/1 -> -2(zeta-lambda)/1
  w_p/1 -> [w_p], Product6/1, Product4/2, Product4/1, Product2/1, Product1/1
  k1/1 -> Product2/2
  Product3/1 -> K1(w_p)/1
  Matrix Concatenation/1 -> Product3/1
  pos_injection/1 -> Product9/2, Product8/2, Product7/2, Product3/2
  Product10/1 -> K2(w_1)/1
  Product9/1 -> K4/1
  I2/1 -> k1/1
  Switch/1 -> Product7/1
  K2_no_waves/1 -> Create Diagonal Matrix2/1
  [w_p] -> Switch/2
  Product2/1 -> Switch/1
  NPO_gains/1 -> Demux/1
  Demux/1 -> Mux4/1
  Demux/2 -> Mux4/2
  Demux/3 -> Mux4/3
  Demux/4 -> Mux5/1
  Demux/5 -> Mux5/2
  Demux/6 -> Mux5/3
  Mux4/1 -> [K3min]
  Mux5/1 -> [K4]
  [K3min] -> Create Diagonal Matrix/1
  Create Diagonal Matrix/1 -> Matrix Multiply/1
  M/1 -> Matrix Multiply/2
  Create Diagonal Matrix1/1 -> Matrix Multiply1/1
  M1/1 -> Matrix Multiply1/2
  Matrix Multiply1/1 -> Product9/1
  [K4] -> Create Diagonal Matrix1/1
  Matrix Multiply/1 -> Product8/1
  Demux/7 -> [scaleK2]
  Product7/1 -> Product10/1
  [scaleK2] -> Product10/2
  Product8/1 -> K3min/1
  Create Diagonal Matrix2/1 -> Switch/3
